simulink model "ComparaisonDes2retours"  (R2015a)
settings: Solver=ode45  StartTime=0.0  StopTime=10.0  RelTol=1e-3
undefined symbols (not defined in the file or in its folder): CommTD, CommTD_integral, EE0
settings Model: Creator=Lucien  LastModifiedBy=Lucien

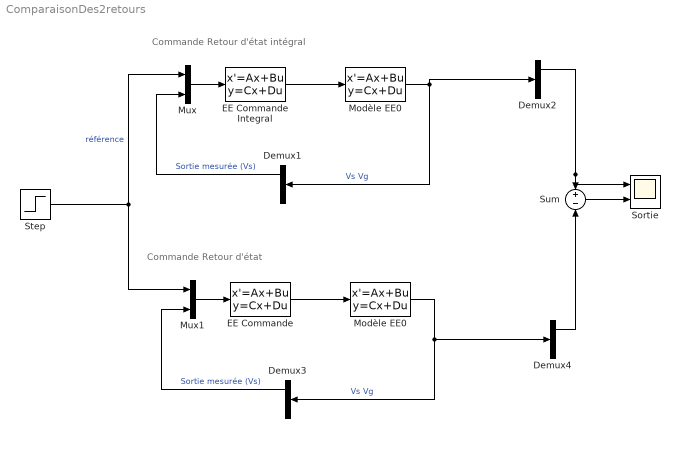
== system ComparaisonDes2retours ==
  note: Commande Retour d'état
  note: Commande Retour d'état intégral
  Demux{1..4} (4 alike) : Demux  Outputs=2
  EE Commande : StateSpace  A=CommTD.ee.a  B=CommTD.ee.b  C=CommTD.ee.c  D=CommTD.ee.d  X0=0
  EE Commande Integral : StateSpace  A=CommTD_integral.ee.a  B=CommTD_integral.ee.b  C=CommTD_integral.ee.c  D=CommTD_integral.ee.d  X0=0
  "Modèle EE0 " : StateSpace  A=EE0.ee.a  B=EE0.ee.b  C=EE0.ee.c  D=EE0.ee.d  X0=0
  "Modèle EE0 " : StateSpace  A=EE0.ee.a  B=EE0.ee.b  C=EE0.ee.c  D=EE0.ee.d  X0=0
  Mux : Mux  Inputs=2
  Mux1 : Mux  Inputs=2
  Sortie : Scope  NumInputPorts=2
      settings: YMin=-5~-5  YMax=5~5  SaveName=ScopeData5
  "Step " : Step  Time=0  SampleTime=0
  Sum : Sum  Inputs=+|-
  wires:
  "Step "/1 -> Mux1/1, Mux/1  "référence"
  EE Commande Integral/1 -> "Modèle EE0 "/1
  Mux/1 -> EE Commande Integral/1
  "Modèle EE0 "/1 -> Demux2/1, Demux1/1  "Vs Vg"
  Demux1/1 -> Mux/2  "Sortie mesurée (Vs)"
  EE Commande/1 -> "Modèle EE0 "/1
  Mux1/1 -> EE Commande/1
  "Modèle EE0 "/1 -> Demux4/1, Demux3/1  "Vs Vg"
  Demux3/1 -> Mux1/2  "Sortie mesurée (Vs)"
  Sum/1 -> Sortie/2
  Demux2/1 -> Sortie/1, Sum/1
  Demux4/1 -> Sum/2
